simulink model "untitled"  (R2020a)
settings: Solver=VariableStepAuto  StartTime=0.0  StopTime=10.0  RelTol=1e-3
undefined symbols (not defined in the file or in its folder): N, PWM
settings Model: Creator=lamarre  LastModifiedBy=lamarre

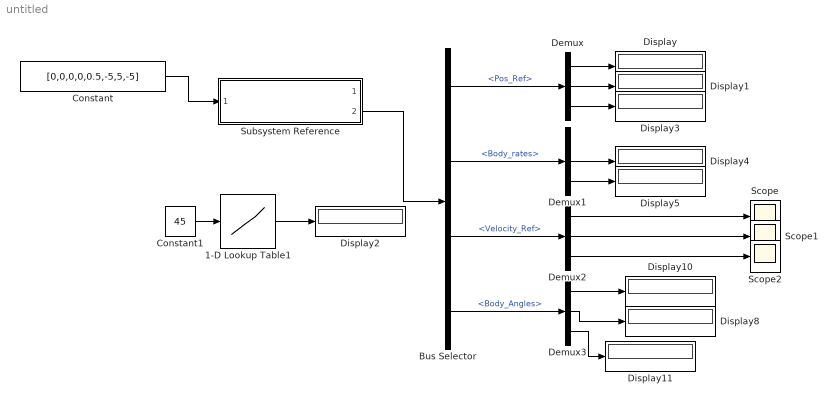
== system untitled ==
  1-D Lookup Table1 : Lookup_n-D  NumberOfTableDimensions=1  BreakpointsForDimension1=N  Table=PWM  InternalRulePriority=Speed  RndMeth=Simplest  InputSameDT=on
  Bus Selector : BusSelector  OutputSignals=Pos_Ref,Body_rates,Velocity_Ref,Body_Angles
  Constant : Constant  Value=[0,0,0,0,0.5,-5,5,-5]
  Constant1 : Constant  Value=45
  Demux{,1..3} (4 alike) : Demux  Outputs=3
  Display{,1..5,8,10..11} (9 alike) : Display
  Scope : Scope
  Scope1 : Scope
  Scope2 : Scope
  Subsystem Reference : Subsystem  ReferencedSubsystem=Plant_and_Environment_Model1
  wires:
  Constant/1 -> Subsystem Reference/1
  Subsystem Reference/2 -> Bus Selector/1
  Bus Selector/1 -> Demux/1  "<Pos_Ref>"
  Bus Selector/2 -> Demux1/1  "<Body_rates>"
  Bus Selector/3 -> Demux2/1  "<Velocity_Ref>"
  Bus Selector/4 -> Demux3/1  "<Body_Angles>"
  Demux/1 -> Display/1
  Demux/2 -> Display1/1
  Demux/3 -> Display3/1
  Demux1/2 -> Display4/1
  Demux1/3 -> Display5/1
  Demux2/1 -> Scope/1
  Demux3/1 -> Display10/1
  Demux3/2 -> Display8/1
  Demux3/3 -> Display11/1
  Demux2/2 -> Scope1/1
  Demux2/3 -> Scope2/1
  Constant1/1 -> 1-D Lookup Table1/1
  1-D Lookup Table1/1 -> Display2/1
